simulink model "project_simulink"  (R2021b)
settings: Solver=VariableStepAuto  StartTime=0.0  StopTime=10e-3  RelTol=1e-3
InitFcn:
  | a = complex(ones(1,21));
undefined symbols (not defined in the file): magnitude
libraries: commfilt2 x6, dspstat3 x5, commrflib2 x2, dspmathops x2
settings Model: Creator=Utente  LastModifiedBy=Utente
settings DataIOCC: ExternalInput=a

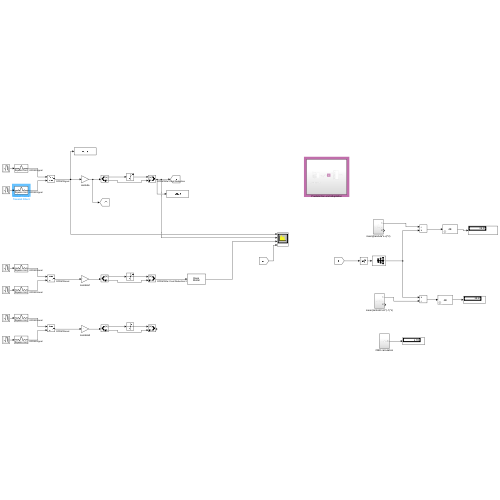
[thumbnail: Simulink's stored preview of the top-level diagram]
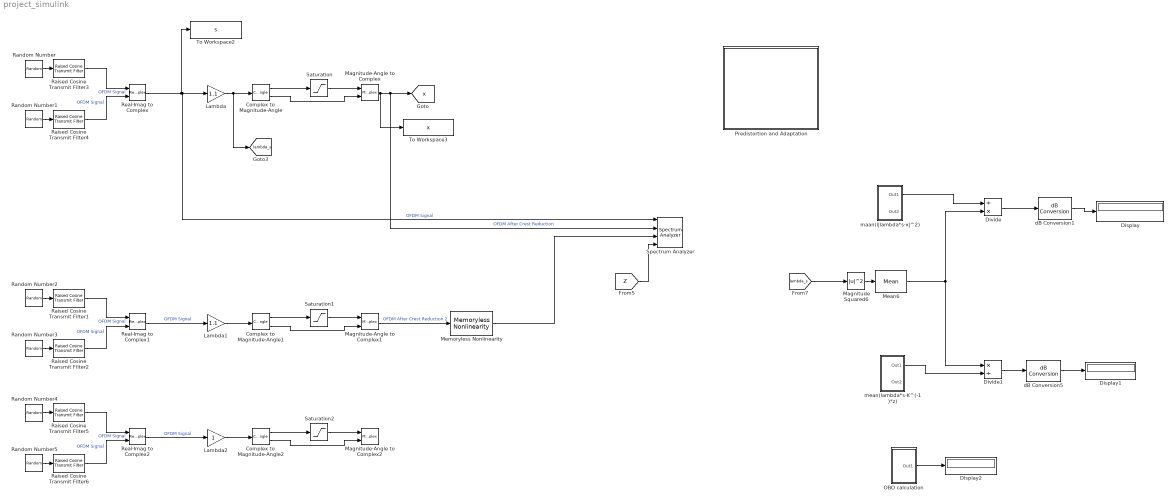
== system project_simulink ==
  Complex to Magnitude-Angle : ComplexToMagnitudeAngle
  Complex to Magnitude-Angle1 : ComplexToMagnitudeAngle
  Complex to Magnitude-Angle2 : ComplexToMagnitudeAngle
  Display : Display
  Display1 : Display
  Display2 : Display
  Divide : Product  Inputs=/*
  Divide1 : Product  Inputs=*/
  Lambda : Gain  Gain=1.1
  Lambda1 : Gain  Gain=1.1
  Lambda2 : Gain
  Magnitude Squared6 : Math  Operator=magnitude^2  SaturateOnIntegerOverflow=on
  Magnitude-Angle to Complex : MagnitudeAngleToComplex
  Magnitude-Angle to Complex1 : MagnitudeAngleToComplex
  Magnitude-Angle to Complex2 : MagnitudeAngleToComplex
  Mean6 : dspstat3/Mean  run=on  reset_popup=None  directionMode=Entire input  dimension=1  roiEnable=off  roiType=Rectangles  roiPortion=Entire ROI  roiOutput=Individual statistics for each ROI  roiFlag=off  roundingMode=Floor  overflowMode=off  outputDataTypeStr=Inherit: Same as accumulator  outputMin=[]  outputMax=[]  outputLastDataTypeStr=Inherit: Same as accumulator
  Memoryless Nonlinearity : commrflib2/Memoryless Nonlinearity  model_select=Rapp model  linGaindB=0  GindB=0  iip3=30  am2pm=10  LPwrLimAMPM=10  UPwrLimAMPM=inf  amam=[2.1587 1.1517]  ampm=[4.0033 9.1040]  x=[8.1081 1.5413 6.5202 -0.0718]  y=[4.6645 2.0965 10.88 -0.003]  p=2  GoutdB=0  vsat=1
      settings: SourceProductBaseCode=CM
  OBO calculation : Subsystem
  Predistortion and Adaptation : Subsystem
  Raised Cosine Transmit Filter1 : commfilt2/Raised Cosine Transmit Filter  filtType=Square root  R=0.2  filtSpan=80  N=8  filterGain=1  RateOptions=Allow multirate processing  framing=Mute  checkCoeff=off  variableName=rcTxFilt1  checkGain=Normalized  sampMode=Mute  saveAsFlag=0  currentFiltSpan=10  D=(10)/2  launchFVT=on  roundingMode=Floor  overflowMode=off  coeffDataTypeStr=Inherit: Same word length as input  coeffMin=[]  coeffMax=[]  coeffLastDataTypeStr=Inherit: Same word length as input  outputDataTypeStr=Inherit: Same as accumulator  outputMin=[]  outputMax=[]  outputLastDataTypeStr=Inherit: Same as accumulator
  Raised Cosine Transmit Filter2 : commfilt2/Raised Cosine Transmit Filter  filtType=Square root  R=0.2  filtSpan=80  N=8  filterGain=1  RateOptions=Allow multirate processing  framing=Mute  checkCoeff=off  variableName=rcTxFilt2  checkGain=Normalized  sampMode=Mute  saveAsFlag=0  currentFiltSpan=10  D=(10)/2  launchFVT=on  roundingMode=Floor  overflowMode=off  coeffDataTypeStr=Inherit: Same word length as input  coeffMin=[]  coeffMax=[]  coeffLastDataTypeStr=Inherit: Same word length as input  outputDataTypeStr=Inherit: Same as accumulator  outputMin=[]  outputMax=[]  outputLastDataTypeStr=Inherit: Same as accumulator
  Raised Cosine Transmit Filter3 : commfilt2/Raised Cosine Transmit Filter  filtType=Square root  R=0.2  filtSpan=80  N=8  filterGain=1  RateOptions=Allow multirate processing  framing=Mute  checkCoeff=off  variableName=rcTxFilt3  checkGain=Normalized  sampMode=Mute  saveAsFlag=0  currentFiltSpan=10  D=(10)/2  launchFVT=on  roundingMode=Floor  overflowMode=off  coeffDataTypeStr=Inherit: Same word length as input  coeffMin=[]  coeffMax=[]  coeffLastDataTypeStr=Inherit: Same word length as input  outputDataTypeStr=Inherit: Same as accumulator  outputMin=[]  outputMax=[]  outputLastDataTypeStr=Inherit: Same as accumulator
  Raised Cosine Transmit Filter4 : commfilt2/Raised Cosine Transmit Filter  filtType=Square root  R=0.2  filtSpan=80  N=8  filterGain=1  RateOptions=Allow multirate processing  framing=Mute  checkCoeff=off  variableName=rcTxFilt4  checkGain=Normalized  sampMode=Mute  saveAsFlag=0  currentFiltSpan=10  D=(10)/2  launchFVT=on  roundingMode=Floor  overflowMode=off  coeffDataTypeStr=Inherit: Same word length as input  coeffMin=[]  coeffMax=[]  coeffLastDataTypeStr=Inherit: Same word length as input  outputDataTypeStr=Inherit: Same as accumulator  outputMin=[]  outputMax=[]  outputLastDataTypeStr=Inherit: Same as accumulator
  Raised Cosine Transmit Filter5 : commfilt2/Raised Cosine Transmit Filter  filtType=Square root  R=0.2  filtSpan=80  N=8  filterGain=1  RateOptions=Allow multirate processing  framing=Mute  checkCoeff=off  variableName=rcTxFilt5  checkGain=Normalized  sampMode=Mute  saveAsFlag=0  currentFiltSpan=10  D=(10)/2  launchFVT=on  roundingMode=Floor  overflowMode=off  coeffDataTypeStr=Inherit: Same word length as input  coeffMin=[]  coeffMax=[]  coeffLastDataTypeStr=Inherit: Same word length as input  outputDataTypeStr=Inherit: Same as accumulator  outputMin=[]  outputMax=[]  outputLastDataTypeStr=Inherit: Same as accumulator
  Raised Cosine Transmit Filter6 : commfilt2/Raised Cosine Transmit Filter  filtType=Square root  R=0.2  filtSpan=80  N=8  filterGain=1  RateOptions=Allow multirate processing  framing=Mute  checkCoeff=off  variableName=rcTxFilt6  checkGain=Normalized  sampMode=Mute  saveAsFlag=0  currentFiltSpan=10  D=(10)/2  launchFVT=on  roundingMode=Floor  overflowMode=off  coeffDataTypeStr=Inherit: Same word length as input  coeffMin=[]  coeffMax=[]  coeffLastDataTypeStr=Inherit: Same word length as input  outputDataTypeStr=Inherit: Same as accumulator  outputMin=[]  outputMax=[]  outputLastDataTypeStr=Inherit: Same as accumulator
  Random Number : RandomNumber  Variance=0.5  Seed=1  SampleTime=0.0000001
  Random Number1 : RandomNumber  Variance=0.5  Seed=2  SampleTime=0.0000001
  Random Number2 : RandomNumber  Variance=0.5  Seed=1  SampleTime=0.0000001
  Random Number3 : RandomNumber  Variance=0.5  Seed=2  SampleTime=0.0000001
  Random Number4 : RandomNumber  Seed=1  SampleTime=0.0000001
  Random Number5 : RandomNumber  Variance=0.5  Seed=2  SampleTime=0.0000001
  Real-Imag to Complex : RealImagToComplex
  Real-Imag to Complex1 : RealImagToComplex
  Real-Imag to Complex2 : RealImagToComplex
  Saturation : Saturate  UpperLimit=1  LowerLimit=0
  Saturation1 : Saturate  UpperLimit=1  LowerLimit=0
  Saturation2 : Saturate  UpperLimit=1  LowerLimit=0
  Spectrum Analyzer : SpectrumAnalyzer  NumInputPorts=4
  To Workspace2 : ToWorkspace  VariableName=s  SampleTime=-1
      settings: Save2DSignal=2-D array (concatenate along first dimension)
  To Workspace3 : ToWorkspace  VariableName=x  SampleTime=-1
      settings: Save2DSignal=2-D array (concatenate along first dimension)
  dB Conversion1 : dspmathops/dB Conversion  dBtype=dB  intype=Power  R=1  fuzz=off
  dB Conversion5 : dspmathops/dB Conversion  dBtype=dB  intype=Power  R=1  fuzz=off
  maan(l|lambda*s-x|^2) : Subsystem
  mean(lambda*s-K^(-1)*z) : Subsystem
  tag scope: lambda_s=global, x=global
  wires:
  Lambda/1 -> [lambda_s], Complex to Magnitude-Angle/1
  Complex to Magnitude-Angle/2 -> Magnitude-Angle to Complex/2
  Saturation/1 -> Magnitude-Angle to Complex/1
  Complex to Magnitude-Angle/1 -> Saturation/1
  Magnitude-Angle to Complex/1 -> To Workspace3/1, Spectrum Analyzer/2, [x]  "OFDM After Crest Reduction"
  Random Number/1 -> Raised Cosine Transmit Filter3/1
  Random Number1/1 -> Raised Cosine Transmit Filter4/1
  Magnitude Squared6/1 -> Mean6/1
  [lambda_s] -> Magnitude Squared6/1
  Mean6/1 -> Divide1/1, Divide/2
  maan(l|lambda*s-x|^2)/1(Out1) -> Divide/1
  mean(lambda*s-K^(-1)*z)/1(Out1) -> Divide1/2
  Divide/1 -> dB Conversion1/1
  Divide1/1 -> dB Conversion5/1
  dB Conversion1/1 -> Display/1
  dB Conversion5/1 -> Display1/1
  OBO calculation/1(Out1) -> Display2/1
  Raised Cosine Transmit Filter4/1 -> Real-Imag to Complex/2  "OFDM Signal"
  Complex to Magnitude-Angle1/1 -> Saturation1/1
  Complex to Magnitude-Angle1/2 -> Magnitude-Angle to Complex1/2
  Random Number2/1 -> Raised Cosine Transmit Filter1/1
  Saturation1/1 -> Magnitude-Angle to Complex1/1
  Raised Cosine Transmit Filter2/1 -> Real-Imag to Complex1/2  "OFDM Signal"
  Lambda1/1 -> Complex to Magnitude-Angle1/1
  Random Number3/1 -> Raised Cosine Transmit Filter2/1
  Complex to Magnitude-Angle2/1 -> Saturation2/1
  Complex to Magnitude-Angle2/2 -> Magnitude-Angle to Complex2/2
  Random Number4/1 -> Raised Cosine Transmit Filter5/1
  Saturation2/1 -> Magnitude-Angle to Complex2/1
  Raised Cosine Transmit Filter6/1 -> Real-Imag to Complex2/2  "OFDM Signal"
  Lambda2/1 -> Complex to Magnitude-Angle2/1
  Random Number5/1 -> Raised Cosine Transmit Filter6/1
  [Z] -> Spectrum Analyzer/4
  Magnitude-Angle to Complex1/1 -> Memoryless Nonlinearity/1  "OFDM After Crest Reduction 2"
  Memoryless Nonlinearity/1 -> Spectrum Analyzer/3
  Raised Cosine Transmit Filter3/1 -> Real-Imag to Complex/1  "OFDM Signal"
  Real-Imag to Complex/1 -> To Workspace2/1, Spectrum Analyzer/1, Lambda/1  "OFDM Signal"
  Raised Cosine Transmit Filter1/1 -> Real-Imag to Complex1/1  "OFDM Signal"
  Real-Imag to Complex1/1 -> Lambda1/1  "OFDM Signal"
  Raised Cosine Transmit Filter5/1 -> Real-Imag to Complex2/1  "OFDM Signal"
  Real-Imag to Complex2/1 -> Lambda2/1  "OFDM Signal"

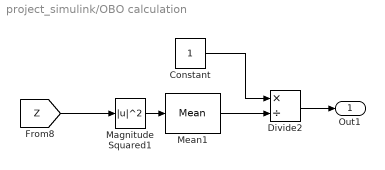
== system project_simulink/OBO calculation ==
  Constant : Constant
  Divide2 : Product  Inputs=*/
  Magnitude Squared1 : Math  Operator=magnitude^2  SaturateOnIntegerOverflow=on
  Mean1 : dspstat3/Mean  run=on  reset_popup=None  directionMode=Entire input  dimension=1  roiEnable=off  roiType=Rectangles  roiPortion=Entire ROI  roiOutput=Individual statistics for each ROI  roiFlag=off  roundingMode=Floor  overflowMode=off  outputDataTypeStr=Inherit: Same as accumulator  outputMin=[]  outputMax=[]  outputLastDataTypeStr=Inherit: Same as accumulator
  Out1 : Outport
  wires:
  Constant/1 -> Divide2/1
  Mean1/1 -> Divide2/2
  [Z] -> Magnitude Squared1/1
  Magnitude Squared1/1 -> Mean1/1
  Divide2/1 -> Out1/1

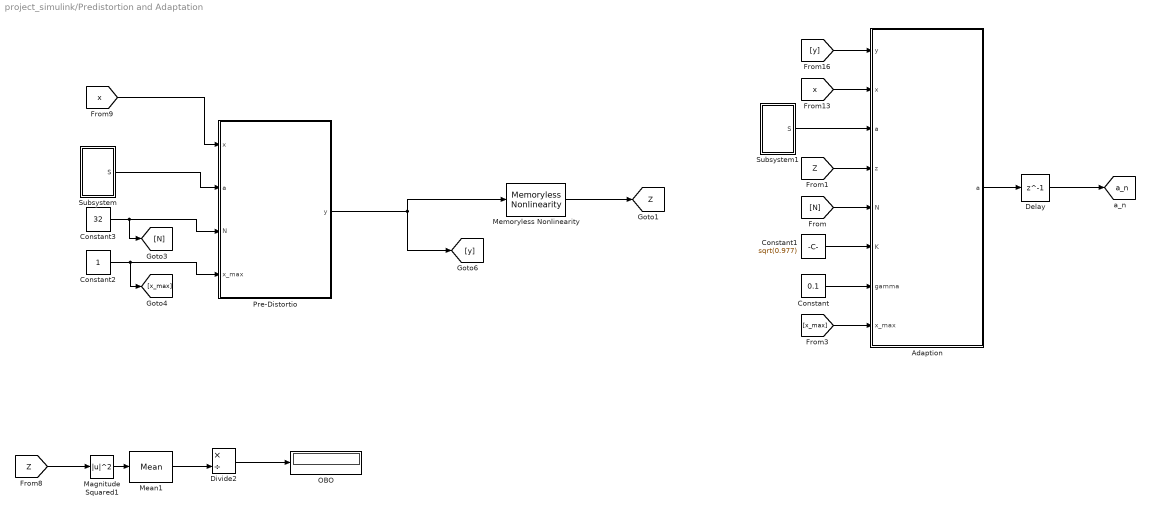
== system project_simulink/Predistortion and Adaptation ==
  "Adaption " : MATLAB Function  TreatAsAtomicUnit=on
  Constant : Constant  Value=0.1
  Constant1 : Constant  Value=sqrt(0.977)
  Constant2 : Constant
  Constant3 : Constant  Value=32
  Delay : Delay  DelayLength=1  InitialCondition=0
  Divide2 : Product  Inputs=*/
  Magnitude Squared1 : Math  Operator=magnitude^2  SaturateOnIntegerOverflow=on
  Mean1 : dspstat3/Mean  run=on  reset_popup=None  directionMode=Entire input  dimension=1  roiEnable=off  roiType=Rectangles  roiPortion=Entire ROI  roiOutput=Individual statistics for each ROI  roiFlag=off  roundingMode=Floor  overflowMode=off  outputDataTypeStr=Inherit: Same as accumulator  outputMin=[]  outputMax=[]  outputLastDataTypeStr=Inherit: Same as accumulator
  Memoryless Nonlinearity : commrflib2/Memoryless Nonlinearity  model_select=Rapp model  linGaindB=0  GindB=0  iip3=30  am2pm=10  LPwrLimAMPM=10  UPwrLimAMPM=inf  amam=[2.1587 1.1517]  ampm=[4.0033 9.1040]  x=[8.1081 1.5413 6.5202 -0.0718]  y=[4.6645 2.0965 10.88 -0.003]  p=2  GoutdB=0  vsat=1
      settings: SourceProductBaseCode=CM
  OBO : Display
  Pre-Distortio : MATLAB Function  TreatAsAtomicUnit=on
  Subsystem : Subsystem
  Subsystem1 : Subsystem
  tag scope: Z=global, a_n=global
  wires:
  [x] -> "Adaption "/2(x)
  "Adaption "/1(a) -> Delay/1
  [x] -> Pre-Distortio/1(x)
  Delay/1 -> [a_n]
  [x_max] -> "Adaption "/8(x_max)
  Constant3/1 -> Pre-Distortio/3(N), [N]
  Pre-Distortio/1(y) -> Memoryless Nonlinearity/1, [y]
  [Z] -> "Adaption "/4(z)
  [y] -> "Adaption "/1(y)
  [N] -> "Adaption "/5(N)
  Constant/1 -> "Adaption "/7(gamma)
  Constant2/1 -> [x_max], Pre-Distortio/4(x_max)
  Constant1/1 -> "Adaption "/6(K)
  Memoryless Nonlinearity/1 -> [Z]
  Subsystem/1(S) -> Pre-Distortio/2(a)
  Subsystem1/1(S) -> "Adaption "/3("a ")
  Magnitude Squared1/1 -> Mean1/1
  Mean1/1 -> Divide2/2
  Divide2/1 -> OBO/1
  [Z] -> Magnitude Squared1/1

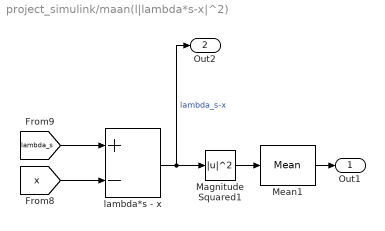
== system project_simulink/maan(l|lambda*s-x|^2) ==
  Magnitude Squared1 : Math  Operator=magnitude^2  SaturateOnIntegerOverflow=on
  Mean1 : dspstat3/Mean  run=on  reset_popup=None  directionMode=Entire input  dimension=1  roiEnable=off  roiType=Rectangles  roiPortion=Entire ROI  roiOutput=Individual statistics for each ROI  roiFlag=off  roundingMode=Floor  overflowMode=off  outputDataTypeStr=Inherit: Same as accumulator  outputMin=[]  outputMax=[]  outputLastDataTypeStr=Inherit: Same as accumulator
  lambda*s - x : Sum  Inputs=+-
  Out1 : Outport
  Out2 : Outport  Port=2
  wires:
  Magnitude Squared1/1 -> Mean1/1
  lambda*s - x/1 -> Out2/1, Magnitude Squared1/1  "lambda_s-x"
  [x] -> lambda*s - x/2
  [lambda_s] -> lambda*s - x/1
  Mean1/1 -> Out1/1

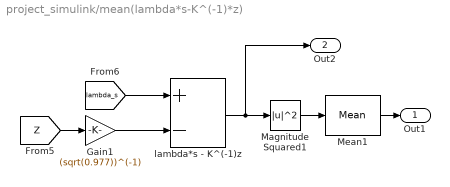
== system project_simulink/mean(lambda*s-K^(-1)*z) ==
  Gain1 : Gain  Gain=(sqrt(0.977))^(-1)
  Magnitude Squared1 : Math  Operator=magnitude^2  SaturateOnIntegerOverflow=on
  Mean1 : dspstat3/Mean  run=on  reset_popup=None  directionMode=Entire input  dimension=1  roiEnable=off  roiType=Rectangles  roiPortion=Entire ROI  roiOutput=Individual statistics for each ROI  roiFlag=off  roundingMode=Floor  overflowMode=off  outputDataTypeStr=Inherit: Same as accumulator  outputMin=[]  outputMax=[]  outputLastDataTypeStr=Inherit: Same as accumulator
  lambda*s - K^(-1)z : Sum  Inputs=+-
  Out1 : Outport
  Out2 : Outport  Port=2
  wires:
  [Z] -> Gain1/1
  Mean1/1 -> Out1/1
  [lambda_s] -> lambda*s - K^(-1)z/1
  Magnitude Squared1/1 -> Mean1/1
  lambda*s - K^(-1)z/1 -> Out2/1, Magnitude Squared1/1
  Gain1/1 -> lambda*s - K^(-1)z/2

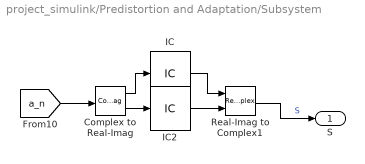
== system project_simulink/Predistortion and Adaptation/Subsystem ==
  Complex to Real-Imag : ComplexToRealImag
  IC : InitialCondition  Value=ones(1,33)
  IC2 : InitialCondition  Value=zeros(1,33)
  Real-Imag to Complex1 : RealImagToComplex
  S : Outport
  wires:
  Complex to Real-Imag/2 -> IC2/1
  IC2/1 -> Real-Imag to Complex1/2
  [a_n] -> Complex to Real-Imag/1
  IC/1 -> Real-Imag to Complex1/1
  Complex to Real-Imag/1 -> IC/1
  Real-Imag to Complex1/1 -> S/1  "S"

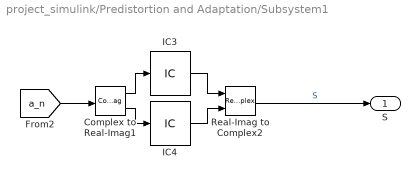
== system project_simulink/Predistortion and Adaptation/Subsystem1 ==
  Complex to Real-Imag1 : ComplexToRealImag
  IC3 : InitialCondition  Value=ones(1,33)
  IC4 : InitialCondition  Value=zeros(1,33)
  Real-Imag to Complex2 : RealImagToComplex
  S : Outport
  wires:
  IC4/1 -> Real-Imag to Complex2/2
  [a_n] -> Complex to Real-Imag1/1
  Real-Imag to Complex2/1 -> S/1  "S"
  Complex to Real-Imag1/2 -> IC4/1
  IC3/1 -> Real-Imag to Complex2/1
  Complex to Real-Imag1/1 -> IC3/1

== matlab function project_simulink/Predistortion and Adaptation/Pre-Distortio ==
  data: x input; y output size=1; a input; N input; x_max input
function y  = predistortion(x,a,N,x_max)
    %Interval detection
    delta = abs(x_max) / (2*N); 
    % All intervals
    I = [delta*2:delta*2:x_max inf];
    % Find the Parameter Index where the abs(x) falls
    n = 1:(N+1);
    n = n(abs(x) < I);
    n = n(1);
    % Piecewise Linear Interpolation
    P_x = ((abs(x) - (2*n-1)*delta) * (a(min(n+1,N+1)) - a(n)) / (2*delta)) + ((a(min(n+1,N+1)) + a(n)) / 2);
    % Output
    y_old = complex( x * P_x);
    y = y_old;
end

== matlab function project_simulink/Predistortion and Adaptation/Adaption  ==
  data: y input; x input; a input; a output; z input; N input; K input; gamma input; x_max input
function a = Adaption(y, x, a, z, N, K, gamma, x_max)
    
    %Re-do the same because of causality of the first initialization
    delta = abs(x_max) / (2*N);
    % All Intervals
    I = [delta:delta*2:x_max inf];
    n = 1:(N+1);
    n = n(abs(x) < I);
    n = n(1);
    % Update Coefficients
    a(n) = (a(n) - gamma * (z - K * x) * conj(z) / conj(y) * conj(x)); 
end
